simulink model "PTODi_TrqLeadCoord"  (R2016b)
settings: configuration reference "CodeGenConfigSet" (kept outside this file)
settings Model: Creator=Wollf  LastModifiedBy=Wollf
settings ConfigSetRef: SourceLocation=Base Workspace

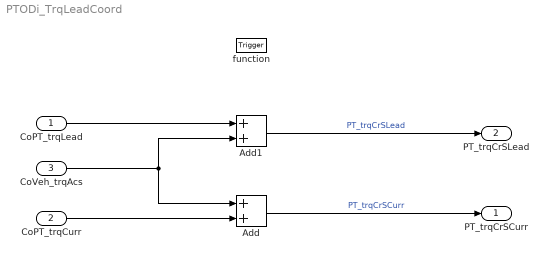
== system PTODi_TrqLeadCoord ==
  CoPT_trqLead : Inport  Tag=Nm  Description=Rate action moment order moment place (Clutch moment)  OutMin=-3000  OutMax=3000  OutDataTypeStr=Trq_Nm
  CoPT_trqCurr : Inport  Tag=Nm  Description=Lead torque order for rail pressure control (clutch torque)  Port=2  OutMin=-3000  OutMax=3000  OutDataTypeStr=Trq_Nm
  CoVeh_trqAcs : Inport  Tag=Nm  Description=message for demand of accessories  Port=3  OutMin=-3276.8  OutMax=3276.7  OutDataTypeStr=Trq_Nm
  function : TriggerPort  TriggerType=function-call  VariantControl=Variant
  Add : Sum  SaturateOnIntegerOverflow=on
  Add1 : Sum  SaturateOnIntegerOverflow=on
  PT_trqCrSCurr : Outport  Tag=Nm  Description=application parameter for lead torque order to engine for rail pressure control（crankshaft torque）  OutMin=-3000  OutMax=3000  OutDataTypeStr=Trq_Nm
  PT_trqCrSLead : Outport  Tag=Nm  Description=application parameter for lead torque order to engine（crankshaft torque）  Port=2  OutMin=-3000  OutMax=3000  OutDataTypeStr=Trq_Nm
  wires:
  CoPT_trqLead/1 -> Add1/1
  CoVeh_trqAcs/1 -> Add/1, Add1/2
  CoPT_trqCurr/1 -> Add/2
  Add1/1 -> PT_trqCrSLead/1  "PT_trqCrSLead"
  Add/1 -> PT_trqCrSCurr/1  "PT_trqCrSCurr"
